simulink model "EHRTC_Equation"  (R2018b)
settings: Solver=VariableStepAuto  StartTime=0.0  StopTime=12000  RelTol=1e-3
undefined symbols (not defined in the file): A, B, C, D
settings Model: Creator=bogda  LastModifiedBy=bogda

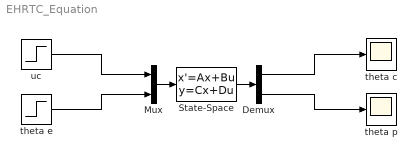
== system EHRTC_Equation ==
  Demux : Demux  Outputs=2
  Mux : Mux  Inputs=2
  State-Space : StateSpace  A=A  B=B  C=C  D=D  InitialCondition=0
  "theta c " : Scope
  theta e : Step  Time=5000  After=-10  SampleTime=0
  theta p : Scope
  uc : Step  Time=0  After=2.5  SampleTime=0
  wires:
  State-Space/1 -> Demux/1
  Mux/1 -> State-Space/1
  uc/1 -> Mux/1
  theta e/1 -> Mux/2
  Demux/1 -> "theta c "/1
  Demux/2 -> theta p/1
